simulink model "Copy_of_Regler"  (R2025b)
settings: Solver=ode23s  StartTime=0  StopTime=100  FixedStep=tStep  RelTol=1e-3  EnableMultiTasking=on
values from neighbouring files (symbols this model uses):
  A = [0 1 0 0 ... (first row only)    [reglerInit.m]    (also in test_init.m; zustandsregler.m)
  B = [0; -30.49; 0; 30.49]    [reglerInit.m]    (also in test_init.m; zustandsregler.m)
  C_new = [1 0 0 0 ... (first row only)    [reglerInit.m]    (also in test_init.m; zustandsregler.m)
  E_temp = zeros(4,12)    [reglerInit.m]    (also in test_init.m)
  G = [1;1;1;1]    [test_init.m]
  Gamma = reshape(gamma_vec,1,4)    [test_init.m]    (also in zustandsregler.m)
  Kx = zeros(6, 4)    [reglerInit.m]    (also in test_init.m)
  Kxi = zeros(6,1)    [reglerInit.m]    (also in test_init.m = zeros(6,4))
  Pi = reshape(pi_vec,4,4)    [test_init.m]    (also in zustandsregler.m)
  Q_sy = [0 1 0 0]    [test_init.m]    (also in zustandsregler.m)
  S_sy = [0 0 0 0 ... (first row only)    [test_init.m]    (also in zustandsregler.m)
  T = 2    [test_init.m]    (also in zustandsregler.m = 50)
  x0 = [0; 0; 1; 0]    [reglerInit.m]    (also in test_init.m = [0; 0; 0; 0]; zustandsregler.m)
  x_soll = -2.45    [test_init.m]
  xi0 = 0    [reglerInit.m]    (also in test_init.m = [0;0;0;0]; zustandsregler.m)
  zhut0 = [0;0;0;0]    [reglerInit.m]    (also in test_init.m; zustandsregler.m)
undefined symbols (not defined in the file or in its folder): ml
settings Model: Creator=Henning Schlüter  LastModifiedBy=marin
settings SolverCC: AlgebraicLoopSolver=TrustRegion
settings DataIOCC: SaveFormat=Array  SignalLoggingSaveFormat=ModelDataLogs  SaveOutput=off  SaveTime=off  ReturnWorkspaceOutputs=off
settings OptimizationCC: ExpressionDepthLimit=2147483647.0  LifeSpan=inf
settings DebuggingCC: UnderspecifiedInitializationDetection=Classic  MergeDetectMultiDrivingBlocksExec=none  SolverPrmCheckMsg=warning  UnconnectedInputMsg=warning  UnconnectedOutputMsg=warning  UnconnectedLineMsg=warning  StateNameClashWarn=warning  PregeneratedLibrarySubsystemCodeDiagnostic=none  SFUnexpectedBacktrackingDiag=warning  SFNoUnconditionalDefaultTransitionDiag=warning  SFExecutionAtInitializationDiag=none  ArithmeticOperatorsInVariantConditions=warning
settings HardwareCC: ProdBitPerPointer=32.0  ProdBitPerSizeT=32.0  ProdBitPerPtrDiffT=32.0  ProdLargestAtomicFloat=None  ProdIntDivRoundTo=Undefined  ProdEndianess=Unspecified  ProdWordSize=32.0  ProdHWDeviceType=32-bit Generic
settings ModelReferenceCC: EnableRefExpFcnMdlSchedulingChecks=on  PropagateSignalLabelsOutOfModel=off
settings SFSimCC: SimUseLocalCustomCode=off  CustomCodeUndefinedFunction=UseInterfaceOnly
settings RTWCC: RTWUseLocalCustomCode=off  GPUComputeCapability=3.5
settings CodeAppCC: StateflowObjectComments=on
settings GRTTargetCC: TargetLangStandard=C89/C90 (ANSI)  CombineOutputUpdateFcns=off  GRTInterface=on
settings ConfigComp: CovMetricSettings=dw  CovSaveCumulativeToWorkspaceVar=on  CovSaveSingleToWorkspaceVar=on  CovExternalEMLEnable=off  CovSFcnEnable=off

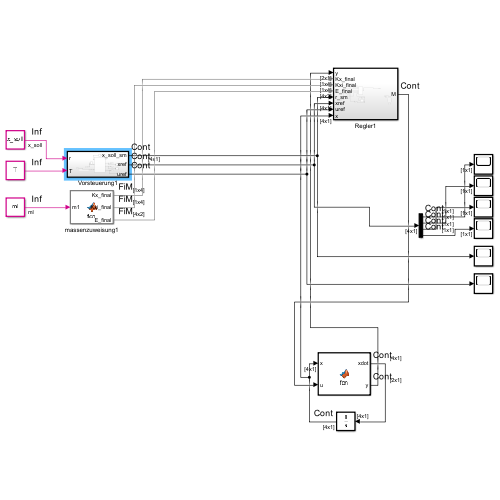
[thumbnail: Simulink's stored preview of the top-level diagram]
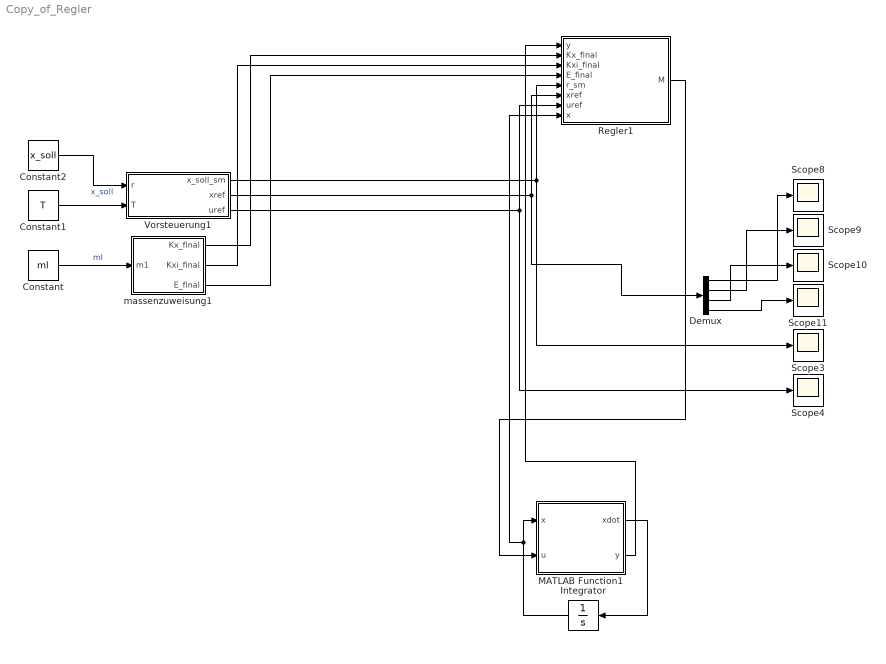
== system Copy_of_Regler ==
  Constant : Constant  Value=ml
  Constant1 : Constant  Value=T
  Constant2 : Constant  Value=x_soll
  Demux : Demux
  Integrator : Integrator  InitialCondition=x0
  MATLAB Function1 : MATLAB Function  TreatAsAtomicUnit=on
  Regler1 : Subsystem
  Scope{3..4,8..11} (6 alike) : Scope
      Scope10 settings: ActiveDisplayYMinimum=-0.10743833551792845  ActiveDisplayYMaximum=0.011937592835327797  DataLoggingVariableName=ScopeData12
      Scope11 settings: ActiveDisplayYMinimum=-0.00060597888158844219  ActiveDisplayYMaximum=6.7330986843160229E-5  DataLoggingVariableName=ScopeData13
      Scope3 settings: ActiveDisplayYMinimum=-0.024999988825888719  ActiveDisplayYMaximum=0.22499989943299853  DataLoggingVariableName=ScopeData3
      Scope4 settings: DataLoggingVariableName=ScopeData6
      Scope8 settings: ActiveDisplayYMinimum=-1.8366370606474449E-7  ActiveDisplayYMaximum=5.3743161431488592E-7  DataLoggingVariableName=ScopeData10
      Scope9 settings: ActiveDisplayYMinimum=-7.163422711585725E-9  ActiveDisplayYMaximum=2.310510206354601E-8  DataLoggingVariableName=ScopeData11
  Vorsteuerung1 : Subsystem
  massenzuweisung1 : MATLAB Function  TreatAsAtomicUnit=on
  wires:
  Demux/1 -> Scope8/1
  Regler1/1(M) -> MATLAB Function1/2(u)
  Vorsteuerung1/2(xref) -> Regler1/6(xref), Demux/1
  Vorsteuerung1/1(x_soll_sm) -> Regler1/5(r_sm), Scope3/1
  massenzuweisung1/2(Kxi_final) -> Regler1/3(Kxi_final)
  MATLAB Function1/2(y) -> Regler1/1(y)
  massenzuweisung1/3(E_final) -> Regler1/4(E_final)
  Demux/4 -> Scope11/1
  Demux/3 -> Scope10/1
  Demux/2 -> Scope9/1
  Constant1/1 -> Vorsteuerung1/2(T)
  massenzuweisung1/1(Kx_final) -> Regler1/2(Kx_final)
  Constant2/1 -> Vorsteuerung1/1(r)  "x_soll"
  Vorsteuerung1/3(uref) -> Regler1/7(uref), Scope4/1
  MATLAB Function1/1(xdot) -> Integrator/1
  Integrator/1 -> Regler1/8(x), MATLAB Function1/1(x)
  Constant/1 -> massenzuweisung1/1(m1)  "ml"

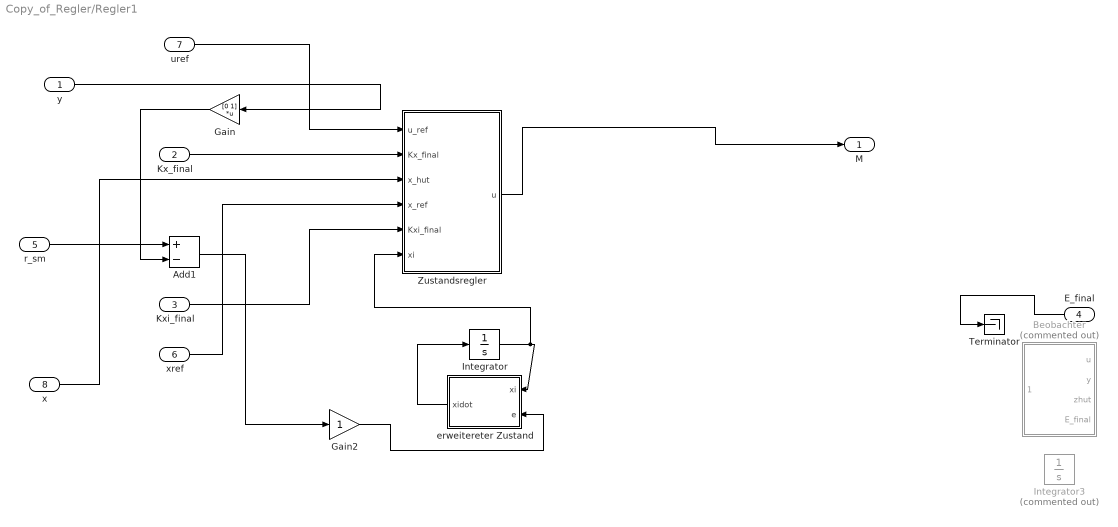
== system Copy_of_Regler/Regler1 ==
  y : Inport
  Kx_final : Inport  Port=2
  Kxi_final : Inport  Port=3
  E_final : Inport  Port=4
  r_sm : Inport  Port=5
  xref : Inport  Port=6
  uref : Inport  Port=7
  x : Inport  Port=8
  Add1 : Sum  Inputs=+-
  Beobachter : MATLAB Function  Commented=on  TreatAsAtomicUnit=on
  Gain : Gain  Gain=[0 1]  Multiplication=Matrix(K*u)
  Gain2 : Gain
  Integrator : Integrator  InitialCondition=xi0
  Integrator3 : Integrator  Commented=on  InitialCondition=zhut0
  Terminator : Terminator
  Zustandsregler : MATLAB Function  TreatAsAtomicUnit=on
  erweitereter Zustand : MATLAB Function  TreatAsAtomicUnit=on
  M : Outport
  wires:
  y/1 -> Gain/1
  Zustandsregler/1(u) -> M/1
  Gain/1 -> Add1/2
  r_sm/1 -> Add1/1
  uref/1 -> Zustandsregler/1(u_ref)
  xref/1 -> Zustandsregler/4(x_ref)
  Kx_final/1 -> Zustandsregler/2(Kx_final)
  Kxi_final/1 -> Zustandsregler/5(Kxi_final)
  erweitereter Zustand/1(xidot) -> Integrator/1
  Integrator/1 -> Zustandsregler/6(xi), erweitereter Zustand/1(xi)
  Gain2/1 -> erweitereter Zustand/2(e)
  Add1/1 -> Gain2/1
  E_final/1 -> Terminator/1
  x/1 -> Zustandsregler/3(x_hut)

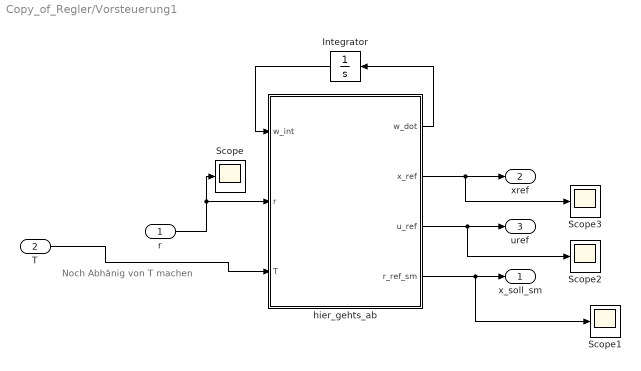
== system Copy_of_Regler/Vorsteuerung1 ==
  note: Noch Abhänig von T machen
  r : Inport
  T : Inport  Port=2
  Integrator : Integrator  InitialCondition=[0;0;0]
  Scope{,1..3} (4 alike) : Scope
      Scope settings: ActiveDisplayYMinimum=0.57263522929680621  ActiveDisplayYMaximum=1.457734004826984  DataLoggingVariableName=ScopeData4
      Scope1 settings: ActiveDisplayYMinimum=-0.15529909957960475  ActiveDisplayYMaximum=0.63159671249896532  DataLoggingVariableName=ScopeData5
      Scope2 settings: ActiveDisplayYMinimum=-0.99801184189333825  ActiveDisplayYMaximum=0.90467258612531509
      Scope3 settings: ActiveDisplayYMinimum=-1.0540214059319417  ActiveDisplayYMaximum=0.82395057453084652
  hier_gehts_ab : MATLAB Function  TreatAsAtomicUnit=on
  x_soll_sm : Outport
  xref : Outport  Port=2
  uref : Outport  Port=3
  wires:
  hier_gehts_ab/1(w_dot) -> Integrator/1
  Integrator/1 -> hier_gehts_ab/1(w_int)
  r/1 -> Scope/1, hier_gehts_ab/2(r)
  hier_gehts_ab/2(x_ref) -> Scope3/1, xref/1
  hier_gehts_ab/3(u_ref) -> Scope2/1, uref/1
  hier_gehts_ab/4(r_ref_sm) -> Scope1/1, x_soll_sm/1
  T/1 -> hier_gehts_ab/3(T)

== matlab function Copy_of_Regler/Vorsteuerung1/hier_gehts_ab ==
  data: w_int input; w_dot output; r input; Pi parameter; Gamma parameter; x_ref output; u_ref output; r_ref_sm output; Q_sy parameter; T input
function [w_dot, x_ref, u_ref, r_ref_sm] = fcn(w_int, r, Pi, Gamma, Q_sy, T)
    % 1. EXPLIZITE GRÖßENZUWEISUNG FÜR DIE AUSGÄNGE (Pre-Allocation)
    % Das bricht den Teufelskreis der Simulink-Größenerkennung am Integrator!
    w_dot = zeros(3, 1);
    x_ref = zeros(4, 1);

    % 2. Eingänge sicher machen
    r_val = double(r(1));                
    T_val = max(double(T(1)), 0.001);    
    w_vec = double(w_int(:));            % Zwingt w_int in einen [3x1] Spaltenvektor
    
    % 3. Workspace-Parameter sicher machen
    Pi_mat = double(Pi);                 
    Gam_vec = double(Gamma(:)');         
    Q_vec = double(Q_sy(:)');            

    % =========================================================
    % 4. Mathematik
    % =========================================================
    A_f = [0, 1, 0; 
           0, 0, 1; 
           -1/(T_val^3), -3/(T_val^2), -3/T_val];
           
    B_f = [0; 0; 1/(T_val^3)];
    
    % 5. Zuweisung in die fest reservierten Variablen
    % Das (:) verbietet Simulink jegliche eigenmächtige Größenänderung!
    w_dot(:) = A_f * w_vec + B_f * r_val;
    
    w = [r_val; w_vec];
    
    x_ref(:) = Pi_mat * w;
    u_ref = Gam_vec * w;
    r_ref_sm = Q_vec * w;
end

== matlab function Copy_of_Regler/massenzuweisung1 ==
  data: m1 input; Kx parameter; Kxi parameter; E_temp parameter; Kx_final output; Kxi_final output; E_final output
function [Kx_final, Kxi_final, E_final]= fcn(m1, Kx, Kxi, E_temp)

E_final = zeros(4,2);
Kx_final = zeros(1,4);
Kxi_final = zeros(1,4);


for i =1:6
    if (m1>i-1 && m1<=i)
        Kx_final = Kx(i,:);
        Kxi_final = Kxi(i,:);
        E_final = E_temp(:,2*i-1:2*i);
    end
end

== matlab function Copy_of_Regler/MATLAB Function1 ==
  data: x input; u input; xdot output; y output; B parameter; A parameter; C_new parameter
function [xdot,y] = fcn(x, u, B, A, C_new)

xdot= A*x+B*u;

y = C_new*x;

== matlab function Copy_of_Regler/Regler1/Beobachter ==
  data: u input; zhutdot output; y input; zhut input; A parameter; B parameter; C_new parameter; E_final input
function zhutdot = fcn(u, y, zhut, A, B, C_new, E_final)


zhutdot = (A-E_final*C_new)*zhut +B*u+E_final*y;

== matlab function Copy_of_Regler/Regler1/Zustandsregler ==
  data: u_ref input; u output; Kx_final input; x_hut input; x_ref input; Kxi_final input; xi input
function u = fcn(u_ref,Kx_final, x_hut, x_ref, Kxi_final,xi)

u = - Kx_final*(x_ref-x_hut)+Kxi_final*xi +  u_ref ;

== matlab function Copy_of_Regler/Regler1/erweitereter Zustand ==
  data: xi input; xidot output; e input; G parameter; S_sy parameter
function xidot = fcn(xi, e, G, S_sy)

Sxi = S_sy;

xidot = Sxi*xi+G*e;
